simulink model "power_estimation"  (R2015a)
settings: Solver=ode3  StartTime=0.0  StopTime=3  FixedStep=Ts  RelTol=1e-3
values from neighbouring files (symbols this model uses):
  Ka = fluxeff    (= 0.15)    [VOC_param.m]    (also in VOC_param_paper.m; power_control_param.m)
  L = 8e-3    (= 0.008)    [VOC_param.m]    (also in VOC_param_paper.m = 0.003; controller_parameters.m = 0.003; current_controller_param.m = 0.005; power_control_param.m = 0.1)
  p = 4    [VOC_param.m]    (also in VOC_param_paper.m; power_control_param.m)
  rpm2radps = pi/30    (= 0.10471975512)    [VOC_param.m]    (also in VOC_param_paper.m; power_control_param.m)
  spq00 = zeros(12,3)    [switch_table_init.m]    (also in switch_table_init1.m; switch_table_init2.m; switch_table_init3.m)
  spq01 = zeros(12,3)    [switch_table_init.m]    (also in switch_table_init1.m; switch_table_init2.m; switch_table_init3.m)
  spq10 = zeros(12,3)    [switch_table_init.m]    (also in switch_table_init1.m; switch_table_init2.m; switch_table_init3.m)
  spq11 = zeros(12,3)    [switch_table_init.m]    (also in switch_table_init1.m; switch_table_init2.m; switch_table_init3.m)
libraries: simulink x1
settings Model: Creator=rblan  LastModifiedBy=rblan

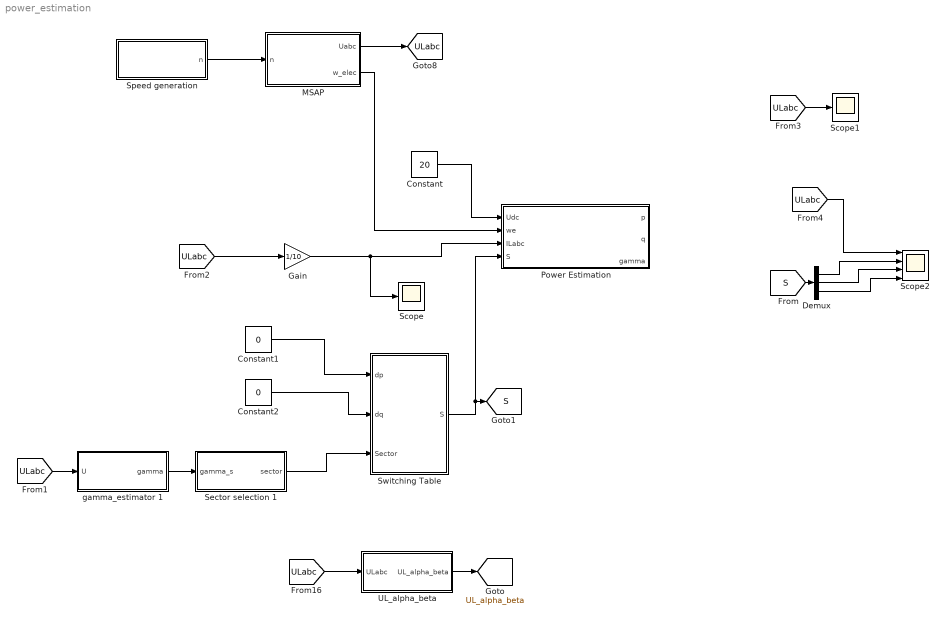
== system power_estimation ==
  Constant : Constant  Value=20
  Constant1 : Constant  Value=0
  Constant2 : Constant  Value=0
  Demux : Demux  Outputs=3
  Gain : Gain  Gain=1/10
  MSAP : Subsystem
  "Power Estimation " : Subsystem
  Scope : Scope
      settings: SaveName=ScopeData5
  Scope1 : Scope
      settings: SaveName=ScopeData8
  Scope2 : Scope  NumInputPorts=4
      settings: YMin=-5~-0.5~-1.5~-1.5  YMax=5~1.5~1.5~1.5  SaveName=ScopeData10
  Sector selection 1 : Subsystem
  Speed generation : Subsystem
  "Switching Table " : Subsystem
  UL_alpha_beta : Subsystem
  gamma_estimator 1 : Subsystem
  tag scope: S=global, UL_alpha_beta=global, ULabc=global
  wires:
  Speed generation/1(n) -> MSAP/1(n)
  [ULabc] -> UL_alpha_beta/1(ULabc)
  UL_alpha_beta/1(UL_alpha_beta) -> [UL_alpha_beta]
  MSAP/1(Uabc) -> [ULabc]
  MSAP/2(w_elec) -> "Power Estimation "/2(we)
  Constant/1 -> "Power Estimation "/1(Udc)
  gamma_estimator 1/1(gamma) -> Sector selection 1/1(gamma_s)
  [ULabc] -> gamma_estimator 1/1(U)
  Constant1/1 -> "Switching Table "/1(dp)
  Constant2/1 -> "Switching Table "/2(dq)
  Sector selection 1/1("sector ") -> "Switching Table "/3("Sector ")
  [ULabc] -> Gain/1
  Gain/1 -> Scope/1, "Power Estimation "/3(ILabc)
  [ULabc] -> Scope1/1
  [ULabc] -> Scope2/1
  "Switching Table "/1(S) -> [S], "Power Estimation "/4(S)
  Demux/2 -> Scope2/3
  Demux/1 -> Scope2/2
  Demux/3 -> Scope2/4
  [S] -> Demux/1

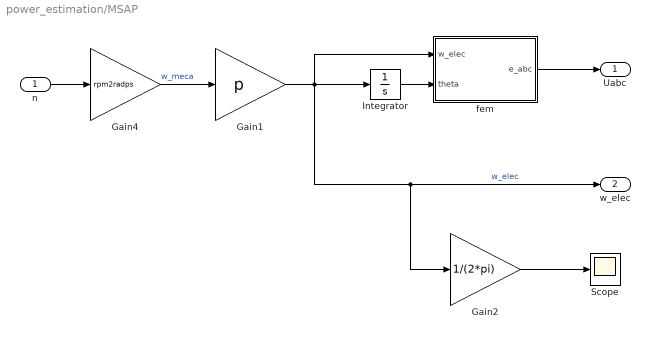
== system power_estimation/MSAP ==
  n : Inport
  Gain1 : Gain  Gain=p
  Gain2 : Gain  Gain=1/(2*pi)
  Gain4 : Gain  Gain=rpm2radps
  Integrator : Integrator
  Scope : Scope
      settings: YMin=19  YMax=21  SaveName=ScopeData9
  fem : Subsystem
  Uabc : Outport
  w_elec : Outport  Port=2
  wires:
  Integrator/1 -> fem/2(theta)
  Gain1/1 -> Integrator/1, Gain2/1, w_elec/1, fem/1(w_elec)  "w_elec"
  n/1 -> Gain4/1
  Gain4/1 -> Gain1/1  "w_meca"
  fem/1(e_abc) -> Uabc/1
  Gain2/1 -> Scope/1

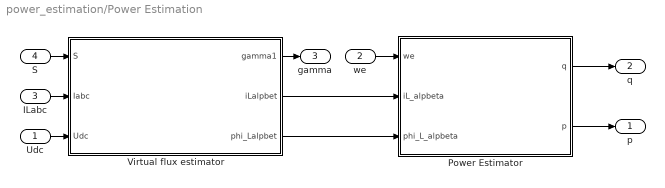
== system power_estimation/Power Estimation  ==
  Udc : Inport
  we : Inport  Port=2
  ILabc : Inport  Port=3
  S : Inport  Port=4
  "Power Estimator " : Subsystem
  Virtual flux estimator : Subsystem
  p : Outport
  q : Outport  Port=2
  gamma : Outport  Port=3
  wires:
  Virtual flux estimator/2(iLalpbet) -> "Power Estimator "/2(iL_alpbeta)
  Virtual flux estimator/3(phi_Lalpbet) -> "Power Estimator "/3(phi_L_alpbeta)
  "Power Estimator "/1(q) -> q/1
  "Power Estimator "/2(p) -> p/1
  S/1 -> Virtual flux estimator/1(S)
  ILabc/1 -> Virtual flux estimator/2(Iabc)
  Udc/1 -> Virtual flux estimator/3(Udc)
  Virtual flux estimator/1(gamma1) -> gamma/1
  we/1 -> "Power Estimator "/1(we)

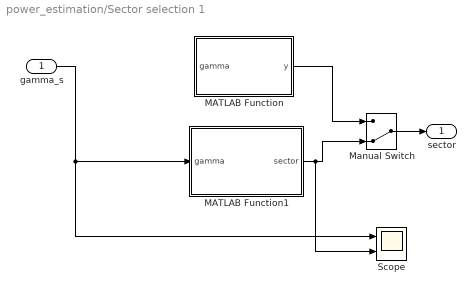
== system power_estimation/Sector selection 1 ==
  gamma_s : Inport
  MATLAB Function : MATLAB Function  TreatAsAtomicUnit=on
  MATLAB Function1 : MATLAB Function  TreatAsAtomicUnit=on
  Manual Switch : ManualSwitch  CurrentSetting=0
  Scope : Scope  NumInputPorts=2
      settings: YMin=0~-5  YMax=6.5~5  SaveName=ScopeData16
  "sector " : Outport
  wires:
  Manual Switch/1 -> "sector "/1
  MATLAB Function1/1(sector) -> Manual Switch/2, Scope/2
  MATLAB Function/1(y) -> Manual Switch/1
  gamma_s/1 -> MATLAB Function1/1(gamma), Scope/1

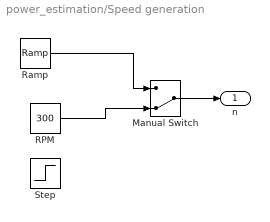
== system power_estimation/Speed generation ==
  Manual Switch : ManualSwitch  CurrentSetting=0
  RPM : Constant  Value=300
  Ramp : simulink/Sources/Ramp  slope=50  start=0  X0=100
  Step : Step  Time=1.5  After=0  SampleTime=0
  n : Outport
  wires:
  Ramp/1 -> Manual Switch/1
  Manual Switch/1 -> n/1
  RPM/1 -> Manual Switch/2

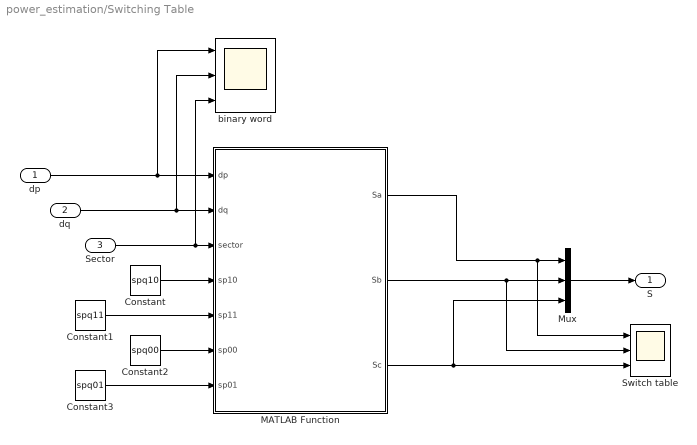
== system power_estimation/Switching Table  ==
  dp : Inport
  dq : Inport  Port=2
  "Sector " : Inport  Port=3
  Constant : Constant  Value=spq10
  Constant1 : Constant  Value=spq11
  Constant2 : Constant  Value=spq00
  Constant3 : Constant  Value=spq01
  MATLAB Function : MATLAB Function  TreatAsAtomicUnit=on
  Mux : Mux  Inputs=3
  Switch table : Scope  NumInputPorts=3
      settings: ShowLegends=on  TimeRange=2  YMin=3~-5~-5  YMax=5~5~5  SaveName=binary_word
  binary word : Scope  NumInputPorts=3
      settings: YMin=-5~-5~-5  YMax=5~5~5  SaveName=ScopeData7
  S : Outport
  wires:
  dp/1 -> binary word/1, MATLAB Function/1(dp)
  "Sector "/1 -> binary word/3, MATLAB Function/3(sector)
  MATLAB Function/2(Sb) -> Switch table/2, Mux/2
  MATLAB Function/3(Sc) -> Mux/3, Switch table/3
  Constant/1 -> MATLAB Function/4(sp10)
  Constant1/1 -> MATLAB Function/5(sp11)
  Constant2/1 -> MATLAB Function/6(sp00)
  Constant3/1 -> MATLAB Function/7(sp01)
  Mux/1 -> S/1
  MATLAB Function/1(Sa) -> Switch table/1, Mux/1
  dq/1 -> binary word/2, MATLAB Function/2(dq)

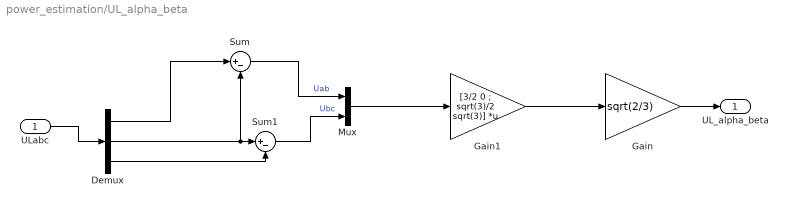
== system power_estimation/UL_alpha_beta ==
  ULabc : Inport
  Demux : Demux  Outputs=3
  Gain : Gain  Gain=sqrt(2/3)
  Gain1 : Gain  Gain=[3/2 0 ; sqrt(3)/2 sqrt(3)]  Multiplication=Matrix(K*u)
  Mux : Mux  Inputs=2
  Sum : Sum  Inputs=|+-
  Sum1 : Sum  Inputs=|+-
  UL_alpha_beta : Outport
  wires:
  ULabc/1 -> Demux/1
  Demux/1 -> Sum/1
  Demux/2 -> Sum/2, Sum1/1
  Demux/3 -> Sum1/2
  Gain/1 -> UL_alpha_beta/1
  Gain1/1 -> Gain/1
  Sum/1 -> Mux/1  "Uab"
  Sum1/1 -> Mux/2  "Ubc"
  Mux/1 -> Gain1/1

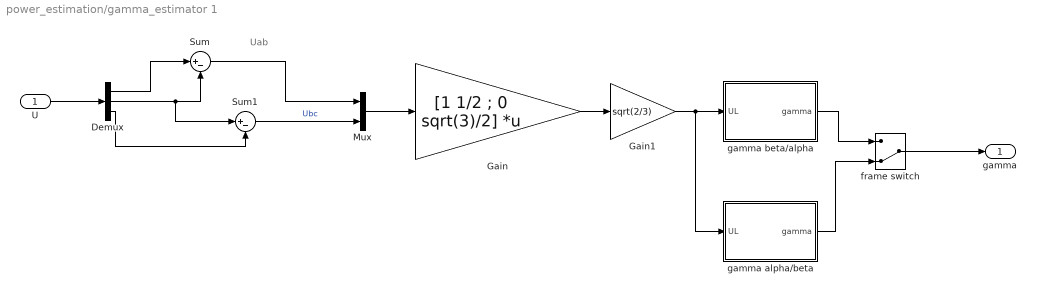
== system power_estimation/gamma_estimator 1 ==
  note: Uab
  U : Inport
  Demux : Demux  Outputs=3
  Gain : Gain  Gain=[1 1/2 ; 0 sqrt(3)/2]  Multiplication=Matrix(K*u)
  Gain1 : Gain  Gain=sqrt(2/3)
  Mux : Mux  Inputs=2
  Sum : Sum  Inputs=|+-
  Sum1 : Sum  Inputs=|+-
  frame switch : ManualSwitch  CurrentSetting=0
  gamma alpha/beta : Subsystem
  gamma beta/alpha : Subsystem
  gamma : Outport
  wires:
  gamma beta/alpha/1(gamma) -> frame switch/1
  frame switch/1 -> gamma/1
  gamma alpha/beta/1(gamma) -> frame switch/2
  Demux/3 -> Sum1/2
  Demux/2 -> Sum/2, Sum1/1
  Demux/1 -> Sum/1
  U/1 -> Demux/1
  Gain1/1 -> gamma beta/alpha/1(UL), gamma alpha/beta/1(UL)
  Sum1/1 -> Mux/2  "Ubc"
  Sum/1 -> Mux/1
  Mux/1 -> Gain/1
  Gain/1 -> Gain1/1

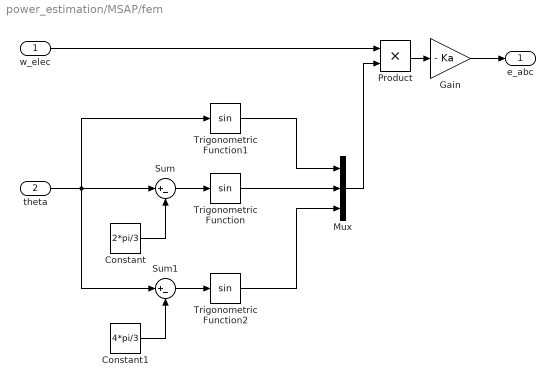
== system power_estimation/MSAP/fem ==
  w_elec : Inport
  theta : Inport  Port=2
  Constant : Constant  Value=2*pi/3
  Constant1 : Constant  Value=4*pi/3
  Gain : Gain  Gain=- Ka
  Mux : Mux  Inputs=3
  Product : Product
  Sum : Sum  Inputs=|+-
  Sum1 : Sum  Inputs=|+-
  Trigonometric Function : Trigonometry
  Trigonometric Function1 : Trigonometry
  Trigonometric Function2 : Trigonometry
  e_abc : Outport
  wires:
  Mux/1 -> Product/2
  theta/1 -> Sum/1, Trigonometric Function1/1, Sum1/1
  Constant1/1 -> Sum1/2
  Sum1/1 -> Trigonometric Function2/1
  Constant/1 -> Sum/2
  Sum/1 -> Trigonometric Function/1
  w_elec/1 -> Product/1
  Product/1 -> Gain/1
  Gain/1 -> e_abc/1
  Trigonometric Function1/1 -> Mux/1
  Trigonometric Function2/1 -> Mux/3
  Trigonometric Function/1 -> Mux/2

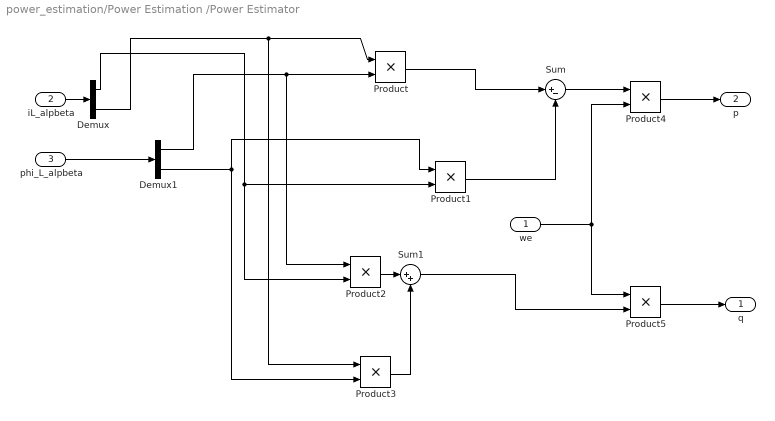
== system power_estimation/Power Estimation /Power Estimator  ==
  we : Inport
  iL_alpbeta : Inport  Port=2
  phi_L_alpbeta : Inport  Port=3
  Demux : Demux  Outputs=2
  Demux1 : Demux  Outputs=2
  Product{,1..5} (6 alike) : Product
  Sum : Sum  Inputs=|+-
  Sum1 : Sum  Inputs=|++
  q : Outport
  p : Outport  Port=2
  wires:
  Product4/1 -> p/1
  Demux1/1 -> Product2/1, Product/2
  Demux/2 -> Product3/1, Product/1
  Product/1 -> Sum/1
  Demux1/2 -> Product3/2, Product1/1
  Demux/1 -> Product2/2, Product1/2
  Product1/1 -> Sum/2
  Product2/1 -> Sum1/1
  Product3/1 -> Sum1/2
  Sum1/1 -> Product5/2
  Product5/1 -> q/1
  iL_alpbeta/1 -> Demux/1
  phi_L_alpbeta/1 -> Demux1/1
  Sum/1 -> Product4/1
  we/1 -> Product5/1, Product4/2

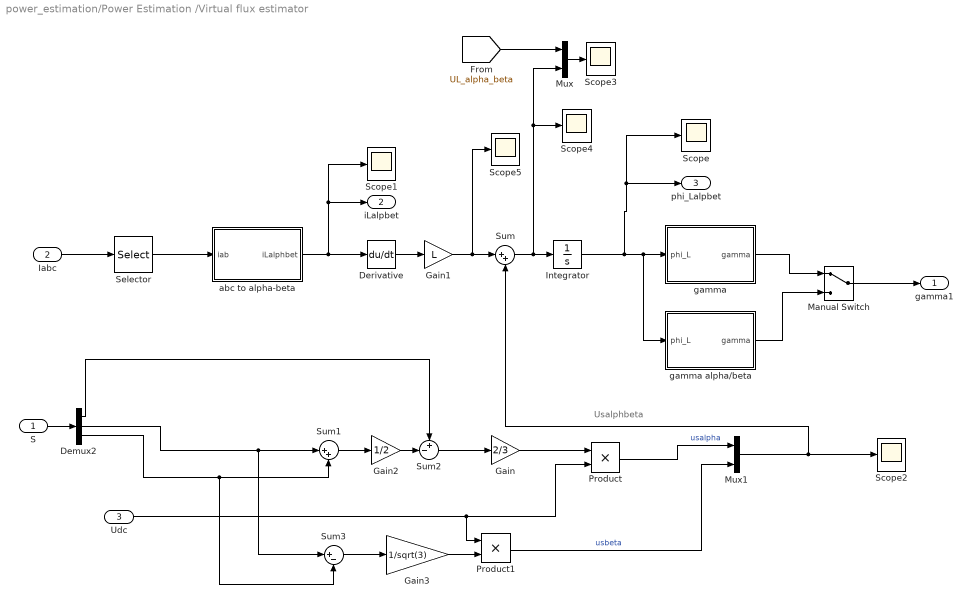
== system power_estimation/Power Estimation /Virtual flux estimator ==
  note: Usalphbeta
  S : Inport
  Iabc : Inport  Port=2
  Udc : Inport  Port=3
  Demux2 : Demux  Outputs=3
  Derivative : Derivative
  Gain : Gain  Gain=2/3
  Gain1 : Gain  Gain=L
  Gain2 : Gain  Gain=1/2
  Gain3 : Gain  Gain=1/sqrt(3)
  Integrator : Integrator
  Manual Switch : ManualSwitch
  Mux : Mux  Inputs=2
  Mux1 : Mux  Inputs=2
  Product : Product
  Product1 : Product
  Scope{,1..5} (6 alike) : Scope
      Scope settings: ShowLegends=on  YMin=-0.45  YMax=0.45
      Scope1 settings: YMin=-450  YMax=450
      Scope2 settings: ShowLegends=on  YMin=-8  YMax=8  SaveName=ScopeData4
      Scope3 settings: ShowLegends=on  YMin=-40  YMax=40  SaveName=ScopeData11
      Scope4 settings: ShowLegends=on  YMin=-40  YMax=40  SaveName=ScopeData6
      Scope5 settings: YMin=-40  YMax=40  SaveName=ScopeData12
  Selector : Selector  InputPortWidth=3  Indices=[1 2]
  Sum : Sum  Inputs=|++
  Sum1 : Sum  Inputs=|++
  Sum2 : Sum  Inputs=+-|
  Sum3 : Sum  Inputs=|+-
  abc to alpha-beta : Subsystem
  gamma : Subsystem
  gamma alpha/beta : Subsystem
  gamma1 : Outport
  iLalpbet : Outport  Port=2
  phi_Lalpbet : Outport  Port=3
  wires:
  abc to alpha-beta/1(iLalphbet) -> Derivative/1, Scope1/1, iLalpbet/1
  Demux2/2 -> Sum3/1, Sum1/1
  Demux2/3 -> Sum3/2, Sum1/2
  Sum1/1 -> Gain2/1
  Gain2/1 -> Sum2/2
  Demux2/1 -> Sum2/1
  Sum2/1 -> Gain/1
  Gain/1 -> Product/1
  Udc/1 -> Product/2, Product1/1
  Product/1 -> Mux1/1  "usalpha"
  Sum3/1 -> Gain3/1
  Gain3/1 -> Product1/2
  Product1/1 -> Mux1/2  "usbeta"
  Integrator/1 -> gamma alpha/beta/1(phi_L), gamma/1(phi_L), Scope/1, phi_Lalpbet/1
  Mux1/1 -> Scope2/1, Sum/2
  S/1 -> Demux2/1
  Selector/1 -> abc to alpha-beta/1(iab)
  Iabc/1 -> Selector/1
  Sum/1 -> Mux/2, Scope4/1, Integrator/1
  Derivative/1 -> Gain1/1
  gamma/1(gamma) -> Manual Switch/1
  gamma alpha/beta/1(gamma) -> Manual Switch/2
  Manual Switch/1 -> gamma1/1
  Mux/1 -> Scope3/1
  [UL_alpha_beta] -> Mux/1
  Gain1/1 -> Scope5/1, Sum/1

== system power_estimation/gamma_estimator 1/gamma alpha//beta ==
  UL : Inport
  Demux : Demux  Outputs=2
  MATLAB Function : MATLAB Function  TreatAsAtomicUnit=on
  Scope2 : Scope  NumInputPorts=2
      settings: TimeRange=10  YMin=-1.75~-500  YMax=1.75~300  SaveName=ScopeData15
  gamma : Outport
  wires:
  MATLAB Function/1(gamma) -> Scope2/2, gamma/1
  Demux/2 -> MATLAB Function/2(beta)  "U_Lbeta"
  Demux/1 -> MATLAB Function/1(alpha)
  UL/1 -> Demux/1, Scope2/1

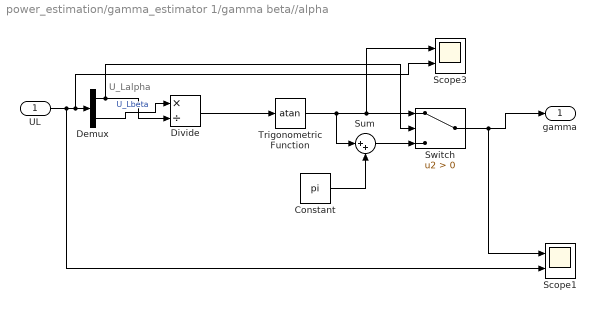
== system power_estimation/gamma_estimator 1/gamma beta//alpha ==
  note: U_Lalpha
  UL : Inport
  Constant : Constant  Value=pi
  Demux : Demux  Outputs=2
  Divide : Product  Inputs=*/
  Scope1 : Scope  NumInputPorts=2
      settings: ShowLegends=on  YMin=-2~-1.25  YMax=5~2  SaveName=ScopeData3
  Scope3 : Scope  NumInputPorts=2
      settings: YMin=-1.75~-500  YMax=1.75~300  SaveName=ScopeData2
  Sum : Sum  Inputs=|++
  Switch : Switch  Criteria=u2 > Threshold
  Trigonometric Function : Trigonometry  Operator=atan
  gamma : Outport
  wires:
  Switch/1 -> gamma/1, Scope1/1
  Sum/1 -> Switch/3
  Trigonometric Function/1 -> Switch/1, Scope3/1, Sum/1
  Divide/1 -> Trigonometric Function/1
  Constant/1 -> Sum/2
  Demux/2 -> Divide/1  "U_Lbeta"
  Demux/1 -> Switch/2, Divide/2
  UL/1 -> Demux/1, Scope3/2, Scope1/2

== system power_estimation/Power Estimation /Virtual flux estimator/abc to alpha-beta ==
  iab : Inport
  Gain : Gain  Gain=sqrt(2/3)
  Gain1 : Gain  Gain=[3/2 0 ; sqrt(3)/2 sqrt(3)]  Multiplication=Matrix(K*u)
  iLalphbet : Outport
  wires:
  Gain1/1 -> Gain/1
  iab/1 -> Gain1/1
  Gain/1 -> iLalphbet/1

== system power_estimation/Power Estimation /Virtual flux estimator/gamma ==
  phi_L : Inport
  Demux : Demux  Outputs=2
  MATLAB Function : MATLAB Function  TreatAsAtomicUnit=on
  Scope1 : Scope  NumInputPorts=2
      settings: ShowLegends=on  YMin=-0.3~0  YMax=0.3~6.5  SaveName=ScopeData3
  gamma : Outport
  wires:
  phi_L/1 -> Scope1/1, Demux/1
  Demux/1 -> MATLAB Function/1(alpha)
  Demux/2 -> MATLAB Function/2(beta)  "phi_Lbeta"
  MATLAB Function/1(gamma) -> Scope1/2, gamma/1

== system power_estimation/Power Estimation /Virtual flux estimator/gamma alpha//beta ==
  phi_L : Inport
  Demux : Demux  Outputs=2
  MATLAB Function : MATLAB Function  TreatAsAtomicUnit=on
  Scope2 : Scope  NumInputPorts=2
      settings: YMin=-1.75~-500  YMax=1.75~300  SaveName=ScopeData15
  gamma : Outport
  wires:
  phi_L/1 -> Scope2/1, Demux/1
  Demux/1 -> MATLAB Function/1(alpha)
  Demux/2 -> MATLAB Function/2(beta)  "phi_Lbeta"
  MATLAB Function/1(gamma) -> gamma/1, Scope2/2

== matlab function power_estimation/Switching Table /MATLAB Function ==
  data: dp input; Sa output; dq input; sector input; Sb output; Sc output; sp10 input; sp11 input; sp00 input; sp01 input
function [Sa,Sb,Sc] = switch_selector(dp,dq,sector,sp10,sp11,sp00,sp01)
%#codegen
% global sp10 sp11 sp00 sp01
% 
% sp10= load('sp10.mat') ; 
% sp11=load('sp11.mat'); 
% sp00=load('sp00.mat');
% sp01 =load('sp01.mat'); 
%persistent Sa Sb Sc  
Sa= 0 ; 
Sb = 0 ; 
Sc = 0 ; 

switch dp
    case 1 
        switch dq
            case 0 
                Sa=sp10(sector,1) ; 
                Sb=sp10(sector,2) ; 
                Sc=sp10(sector,3) ; 
            case 1 
                Sa=sp11(sector,1) ; 
                Sb=sp11(sector,2) ; 
                Sc=sp11(sector,3) ; 
        end
    case 0 
        switch dq
            case 0 
                Sa=sp00(sector,1) ; 
                Sb=sp00(sector,2) ; 
                Sc=sp00(sector,3) ; 
            case 1 
                Sa=sp01(sector,1) ; 
                Sb=sp01(sector,2) ; 
                Sc=sp01(sector,3) ; 
        end
        
end

== matlab function power_estimation/Power Estimation /Virtual flux estimator/gamma/MATLAB Function ==
  data: alpha input; gamma output; beta input
function gamma = gamma_estimator(alpha,beta)
%#codegen

gamma = 0 ; 
gamma = atan(beta/alpha)+pi/2 ; 

if (alpha<0 )
    gamma = gamma +pi ; 
end 

if (beta<0 && alpha> 0 ) 
    gamma = gamma +2*pi ; 
end 

if (gamma>(2*pi) )
    gamma = gamma -2*pi ; 
end

== matlab function power_estimation/Power Estimation /Virtual flux estimator/gamma alpha//beta/MATLAB Function ==
  data: alpha input; gamma output; beta input
function gamma = gamma_estimator(alpha,beta)
%#codegen

gamma = 0 ; 
gamma = atan(beta/alpha) ; 

if (alpha<0 )
    gamma = gamma +pi ; 
end 

if (beta<0 && alpha> 0 ) 
    gamma = gamma +2*pi ; 
end

== matlab function power_estimation/Sector selection 1/MATLAB Function ==
  data: gamma input; y output
function y = fcn(gamma)
%#codegen

% persistent n ; 
% n = 1 ; 
% 
% % gamma
% up = (n-1)*pi/6  ; 
% down = (n-2)*pi/6 ;  
% % n 
% 
% 
% if (n>=11 && gamma <0 ) 
%     gamma = gamma + 2*pi ; 
% end 
% while (down >=gamma || gamma > up) 
%     if n==12 
%         n=1 ; 
%     else 
%         n=n+1  
%     end
%    if (n>=11 && gamma <0 ) 
%     gamma = gamma + 2*pi ; 
%    end 
%     up = (n-1)*pi/6  
%     down = (n-2)*pi/6 
%     gamma
% end 
% y=n 


% gamma
if (gamma < -pi/6) 
    gamma = gamma +2*pi ; 
end 
n= 1 ; 
up = (n-1)*pi/6  ; 
down = (n-2)*pi/6 ;  
 
while (down >=gamma || gamma > up) 
    if n==12 
        n=1 ; 
    else 
        n=n+1 ; 
    end
    up = (n-1)*pi/6  ;
    down = (n-2)*pi/6 ;
end 
y=n ;

== matlab function power_estimation/Sector selection 1/MATLAB Function1 ==
  data: gamma input; sector output
function sector = sector_selection(gamma)
%codegen



if (gamma < -pi/6)
    gamma = gamma +2*pi ;
end

n= 1 ;
up = n*pi/6  ;
down = (n-1)*pi/6 ;

while (down >=gamma || gamma > up)
    if n==12
        n=1 ;
    else
        n=n+1 ;
    end
    
    up = n*pi/6  ;
    down = (n-1)*pi/6 ;
end
sector=n ;

== matlab function power_estimation/gamma_estimator 1/gamma alpha//beta/MATLAB Function ==
  data: alpha input; gamma output; beta input
function gamma = gamma_estimator(alpha,beta)
%#codegen

gamma = 0 ; 
gamma = atan(beta/alpha) ; 

if (alpha<0 )
    gamma = gamma +pi ; 
end 

if (beta<0 && alpha> 0 ) 
    gamma = gamma +2*pi ; 
end
